simulink model "Grades"  (R2021a)
settings: Solver=FixedStepDiscrete  StartTime=0.0  StopTime=10.0  RelTol=1e-3  EnableMultiTasking=on
settings Model: Creator=Mina  LastModifiedBy=Mina
settings DataIOCC: ReturnWorkspaceOutputs=off
settings OptimizationCC: DefaultParameterBehavior=Inlined  InlineInvariantSignals=on  EnableMemcpy=off  LifeSpan=1  EfficientTunableParamExpr=on
settings DebuggingCC: UnderspecifiedInitializationDetection=Classic  MergeDetectMultiDrivingBlocksExec=none  SFMachineParentedDataDiag=warning  ArithmeticOperatorsInVariantConditions=warning
settings ModelReferenceCC: PropagateSignalLabelsOutOfModel=off
settings SFSimCC: MATLABDynamicMemAlloc=off  CustomCodeUndefinedFunction=UseInterfaceOnly
settings RTWCC: SystemTargetFile=ert.tlc  GenCodeOnly=on  TemplateMakefile=ert_default_tmf  GenerateReport=on  IncludeHyperlinkInReport=on  LaunchReport=on  GenerateTraceInfo=on  GenerateTraceReport=on  GenerateTraceReportSl=on  GenerateTraceReportSf=on  GenerateTraceReportEml=on
settings CodeAppCC: ForceParamTrailComments=on  IgnoreCustomStorageClasses=off  OperatorAnnotations=on  SimulinkDataObjDesc=on  SFDataObjDesc=on  MATLABFcnDesc=on  InsertBlockDesc=on  StateflowObjectComments=on  MATLABSourceComments=on
settings ERTTargetCC: MultiwordLength=2048  GenerateSampleERTMain=on  InlinedParameterPlacement=NonHierarchical  ERTCustomFileTemplate=example_file_process.tlc

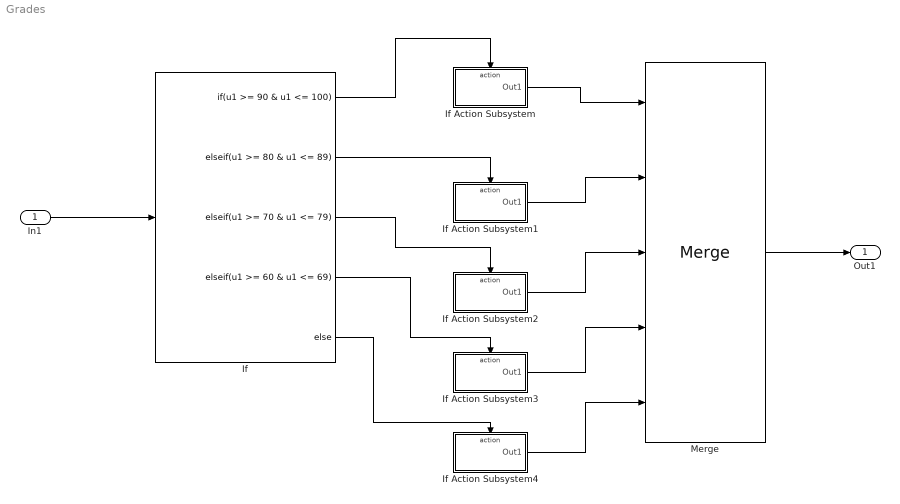
== system Grades ==
  In1 : Inport
  If : If  IfExpression=u1 >= 90 & u1 <= 100  ElseIfExpressions=u1 >= 80 & u1 <= 89 , u1 >= 70 & u1 <= 79 , u1 >= 60 & u1 <= 69
  If Action Subsystem : Subsystem  TreatAsAtomicUnit=on
  If Action Subsystem1 : Subsystem  TreatAsAtomicUnit=on
  If Action Subsystem2 : Subsystem  TreatAsAtomicUnit=on
  If Action Subsystem3 : Subsystem  TreatAsAtomicUnit=on
  If Action Subsystem4 : Subsystem  TreatAsAtomicUnit=on
  Merge : Merge  Inputs=5
  Out1 : Outport
  wires:
  In1/1 -> If/1
  If/1 -> If Action Subsystem/Action
  If/2 -> If Action Subsystem1/Action
  If/3 -> If Action Subsystem2/Action
  If/4 -> If Action Subsystem3/Action
  If/5 -> If Action Subsystem4/Action
  If Action Subsystem/1(Out1) -> Merge/1
  If Action Subsystem1/1(Out1) -> Merge/2
  If Action Subsystem2/1(Out1) -> Merge/3
  If Action Subsystem3/1(Out1) -> Merge/4
  If Action Subsystem4/1(Out1) -> Merge/5
  Merge/1 -> Out1/1

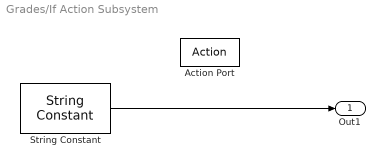
== system Grades/If Action Subsystem ==
  Action Port : ActionPort  ActionPortLabel=if(u1 >= 90 & u1 <= 100)
  String Constant : StringConstant  String="\" Your Grade is A \""
  Out1 : Outport
  wires:
  String Constant/1 -> Out1/1

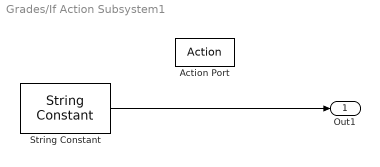
== system Grades/If Action Subsystem1 ==
  Action Port : ActionPort  ActionPortLabel=elseif(u1 >= 80 & u1 <= 89 )
  String Constant : StringConstant  String="\" Your Grade is B \""
  Out1 : Outport
  wires:
  String Constant/1 -> Out1/1

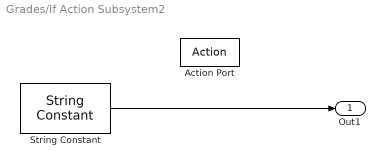
== system Grades/If Action Subsystem2 ==
  Action Port : ActionPort  ActionPortLabel=elseif( u1 >= 70 & u1 <= 79 )
  String Constant : StringConstant  String="\" Your Grade is C \""
  Out1 : Outport
  wires:
  String Constant/1 -> Out1/1

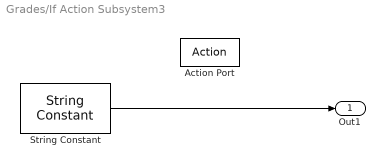
== system Grades/If Action Subsystem3 ==
  Action Port : ActionPort  ActionPortLabel="elseif( u1 >= 60 & u1 <= 69  )"
  String Constant : StringConstant  String="\" Your Grade is D \""
  Out1 : Outport
  wires:
  String Constant/1 -> Out1/1

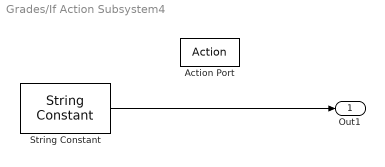
== system Grades/If Action Subsystem4 ==
  Action Port : ActionPort  ActionPortLabel=else
  String Constant : StringConstant  String="\" Your Grade is F \""
  Out1 : Outport
  wires:
  String Constant/1 -> Out1/1
